simulink model "charakterystyki"  (R2019a)
settings: Solver=VariableStepAuto  StartTime=0.0  StopTime=500  RelTol=1e-30
settings Model: Creator=ASUS_PEPE  LastModifiedBy=ASUS_PEPE

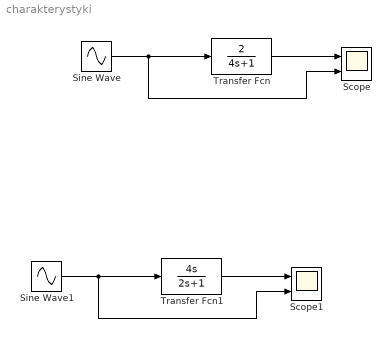
== system charakterystyki ==
  Scope : Scope  NumInputPorts=2
  Scope1 : Scope  NumInputPorts=2
  Sine Wave : Sin  SampleTime=0
  Sine Wave1 : Sin  Frequency=0.1  SampleTime=0
  Transfer Fcn : TransferFcn  Numerator=[2]  Denominator=[4 1]
  Transfer Fcn1 : TransferFcn  Numerator=[4 0]  Denominator=[2 1]
  wires:
  Sine Wave/1 -> Scope/2, Transfer Fcn/1
  Transfer Fcn/1 -> Scope/1
  Transfer Fcn1/1 -> Scope1/1
  Sine Wave1/1 -> Scope1/2, Transfer Fcn1/1
